simulink model "simulacionesTarea7"  (R2021a)
settings: Solver=VariableStepAuto  StartTime=0.0  StopTime=20  RelTol=1e-3
values from neighbouring files (symbols this model uses):
  A = double(A)    [p1p2.m]    (also in p3.m = [-0.8468   -0.0005;54.4218   -7.6617]; p4Discreto1.m = poly2sym(A, z); p5.m = poly2sym(A, z))
  B = double(B)    [p1p2.m]    (also in p3.m = [0;8.3264]; p4Discreto1.m = poly2sym(B, z); p5.m = poly2sym(B, z))
  C = double(C)    [p1p2.m]    (also in p3.m = [0 1])
  denPID = PIDz.den{1}    [P4.m]
  gdzd = Gd.den{1}    [p4Discreto1.m]    (also in p5.m)
  gdzn = Gd.num{1}    [p4Discreto1.m]    (also in p5.m)
  k1 = eval(Sol.k1)    [p3.m]
  k2 = eval(Sol.k2)    [p3.m]
  kc = double(kc)    [experimentoCompensadores.m]    (also in p5compensador.m)
  kd = eval(S.kd)    [P4.m]
  ki = eval(S.ki)    [P4.m]    (also in p3.m = eval(Sol.ki))
  kp = eval(S.kp)    [P4.m]
  L = [PDO(3)-(6.513); PDO(2)-8.508]    [p3.m]
  numPID = PIDz.num{1}    [P4.m]
  r0 = double(vpa(r0))    [p4Discreto1.m]    (also in p5.m)
  s0 = double(vpa(s0))    [p4Discreto1.m]    (also in p5.m)
  s1 = double(vpa(s1))    [p4Discreto1.m]    (also in p5.m)
  s2 = double(vpa(s2))    [p4Discreto1.m]    (also in p5.m)
  tm = 6/300    (= 0.02)    [P4.m]    (also in p4Discreto1.m; p5.m = 0.125)
  UbiCero = double(UbiCero)    [experimentoCompensadores.m]    (also in p5compensador.m)
  UbiPolo = double(UbiPolo)    [experimentoCompensadores.m]    (also in p5compensador.m)
libraries: simulink x2
settings Model: Creator=Cx001la  LastModifiedBy=Cx001la
settings SolverCC: AlgebraicLoopSolver=TrustRegion
settings DataIOCC: ReturnWorkspaceOutputs=off
settings DebuggingCC: SFMachineParentedDataDiag=warning  ArithmeticOperatorsInVariantConditions=warning
settings SFSimCC: SimUseLocalCustomCode=off  CustomCodeUndefinedFunction=UseInterfaceOnly
settings RTWCC: RTWUseLocalCustomCode=off

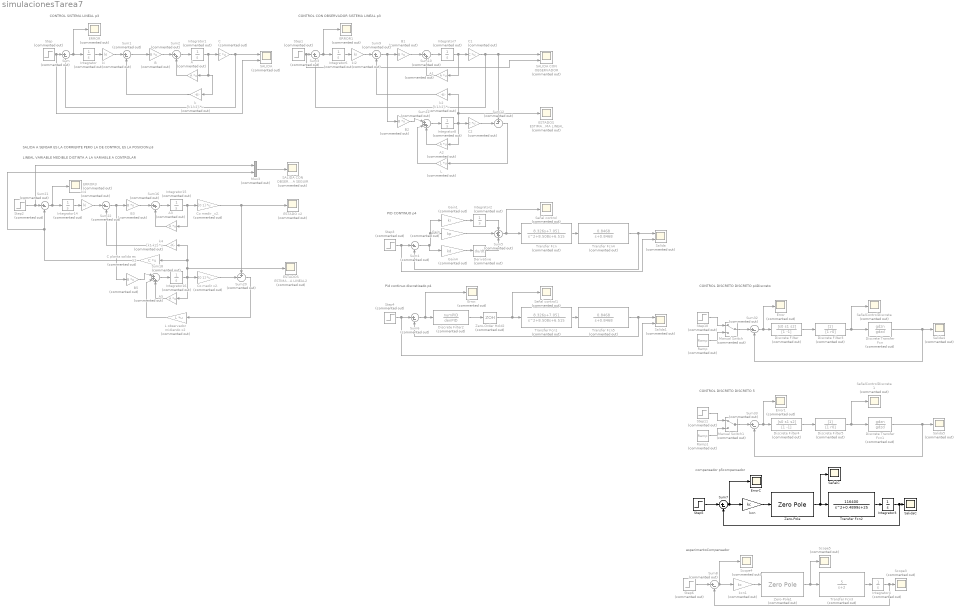
== system simulacionesTarea7 ==
  note: compensador p5compensador
  note: Pid continuo discretizado p4
  note: PID CONTINUO p4
  note: CONTROL SISTEMA LINEAL p3
  note: CONTROL CON OBSERVADOR SISTEMA LINEAL p3
  note: SALIDA A SENSAR ES LA CORRIENTE PERO LA DE CONTROL ES LA POSICION p3
  note: LINEAL VARIABLE MEDIBLE DISTINTA A LA VARIABLE A CONTROLAR
  note: CONTROL DISCRETO DISCRETO p4Discreto
  note: CONTROL DISCRETO DISCRETO 5
  note: esperimentoCompensador
  A{,1..3,5} (5 alike) : Gain  Commented=on  Gain=A  Multiplication=Matrix(K*u)
  B{,1..3,5} (5 alike) : Gain  Commented=on  Gain=B  Multiplication=Matrix(K*u)
  C : Gain  Commented=on  Gain=C  Multiplication=Matrix(K*u)
  C planta salida es X2 : Gain  Commented=on  Gain=C  Multiplication=Matrix(K*u)
  C1 : Gain  Commented=on  Gain=C  Multiplication=Matrix(K*u)
  C2 : Gain  Commented=on  Gain=C  Multiplication=Matrix(K*u)
  Co medir _x2. : Gain  Commented=on  Gain=[0 1]  Multiplication=Matrix(K*u)
  Co medir x2. : Gain  Commented=on  Gain=[0 1]  Multiplication=Matrix(K*u)
  Derivative : Derivative  Commented=on
  Discrete Transfer Fcn : DiscreteTransferFcn  Commented=on  Numerator=gdzn  Denominator=gdzd
  Discrete Transfer Fcn1 : DiscreteTransferFcn  Commented=on  Numerator=gdzn  Denominator=gdzd
  Discrete Filter : DiscreteFilter  Commented=on  Numerator=[s0 s1 s2]  Denominator=[1 -1]
  Discrete Filter2 : DiscreteFilter  Commented=on  Numerator=numPID  Denominator=denPID  SampleTime=tm
  Discrete Filter3 : DiscreteFilter  Commented=on  Denominator=[1 r0]
  Discrete Filter4 : DiscreteFilter  Commented=on  Numerator=[s0 s1 s2]  Denominator=[1 -1]  SampleTime=tm
  Discrete Filter5 : DiscreteFilter  Commented=on  Denominator=[1 r0]  SampleTime=tm
  ERROR : Scope  Commented=on
  ERROR1 : Scope  Commented=on
  ERROR3 : Scope  Commented=on
  ESTADO x2 : Scope  Commented=on
  ESTADOS ESTIMADOS SISTEMA LINEAL : Scope  Commented=on
  ESTADOS ESTIMADOS SISTEMA LINEAL2 : Scope  Commented=on
  Error : Scope  Commented=on
  Error. : Scope  Commented=on
  Error1 : Scope  Commented=on
  ErrorC : Scope
  Gain : Gain  Commented=on  Gain=kp
  Gain1 : Gain  Commented=on  Gain=ki
  Gain4 : Gain  Commented=on  Gain=kd
  Integrator{,1..2,4,6..8,14..16} (10 alike) : Integrator  Commented=on
  Integrator3 : Integrator
  L : Gain  Commented=on  Gain=L  Multiplication=Matrix(K*u)
  L observador midiendo x2 : Gain  Commented=on  Gain=L  Multiplication=Matrix(K*u)
  Manual Switch : ManualSwitch  Commented=on
  Manual Switch1 : ManualSwitch  Commented=on
  Mux3 : Mux  Commented=on  Inputs=2
  Ramp : simulink/Sources/Ramp  Commented=on  slope=1  start=0  InitialOutput=0
  Ramp1 : simulink/Sources/Ramp  Commented=on  slope=1  start=0  InitialOutput=0
  SALIDA : Scope  Commented=on  NumInputPorts=2
  "SALIDA CON OBSERVADOR " : Scope  Commented=on  NumInputPorts=2
  SALIDA CON OBSERVADOR SALIDA ESTIMADA VS REFERENCIA A SEGUIR : Scope  Commented=on
  Salida : Scope  Commented=on  NumInputPorts=2
  Salida1 : Scope  Commented=on  NumInputPorts=2
  Salida4 : Scope  Commented=on
  Salida5 : Scope  Commented=on
  SalidaC : Scope
  Scope3 : Scope  Commented=on
  Scope4 : Scope  Commented=on
  Scope5 : Scope  Commented=on
  Señal control : Scope  Commented=on
  Señal control1 : Scope  Commented=on
  SeñalC : Scope
  SeñalControlDiscreta : Scope  Commented=on
  SeñalControlDiscreta1 : Scope  Commented=on
  Step{,1..2,4,6,11} (6 alike) : Step  Commented=on  Time=0  SampleTime=0
  Step10 : Step  Commented=on  SampleTime=0
  Step3 : Step  Commented=on  SampleTime=0
  Step5 : Step  Time=0  SampleTime=0
  Sum{,1,3..4,6,8..9,21..22,32..33} (11 alike) : Sum  Commented=on  Inputs=|+-
  Sum10 : Sum  Commented=on  Inputs=|++
  Sum11 : Sum  Commented=on  Inputs=|+++
  Sum12 : Sum  Commented=on  Inputs=+-|
  Sum16 : Sum  Commented=on  Inputs=|++
  Sum18 : Sum  Commented=on  Inputs=|+++
  Sum2 : Sum  Commented=on  Inputs=|++
  Sum20 : Sum  Commented=on  Inputs=+-|
  Sum5 : Sum  Commented=on  Inputs=+++
  Sum7 : Sum  Inputs=|+-
  Transfer Fcn : TransferFcn  Commented=on  Numerator=[8.326 7.051]  Denominator=[1 8.508 6.515]
  Transfer Fcn1 : TransferFcn  Commented=on  Numerator=[8.326 7.051]  Denominator=[1 8.508 6.515]
  Transfer Fcn2 : TransferFcn  Numerator=[116400]  Denominator=[1 0.4899 25]
  Transfer Fcn3 : TransferFcn  Commented=on  Numerator=[5]  Denominator=[1 2]
  Transfer Fcn4 : TransferFcn  Commented=on  Numerator=[0.8468]  Denominator=[1 0.8468]
  Transfer Fcn5 : TransferFcn  Commented=on  Numerator=[0.8468]  Denominator=[1 0.8468]
  Zero-Order Hold2 : ZeroOrderHold  Commented=on  SampleTime=tm
  Zero-Pole : ZeroPole  Zeros=[-UbiCero]  Poles=[-UbiPolo]
  Zero-Pole1 : ZeroPole  Commented=on  Zeros=[-UbiCero]  Poles=[-UbiPolo]
  k : Gain  Commented=on  Gain=[k1 k2]  Multiplication=Matrix(K*u)
  k2 : Gain  Commented=on  Gain=[k1 k2]  Multiplication=Matrix(K*u)
  k4 : Gain  Commented=on  Gain=[k1 k2]  Multiplication=Matrix(K*u)
  kcn : Gain  Gain=kc
  kcn1 : Gain  Commented=on  Gain=kc
  ki : Gain  Commented=on  Gain=ki
  ki2 : Gain  Commented=on  Gain=ki
  ki4 : Gain  Commented=on  Gain=ki
  wires:
  C2/1 -> Sum12/2
  Sum3/1 -> ERROR1/1, Integrator6/1
  A/1 -> Sum2/2
  Sum/1 -> ERROR/1, Integrator/1
  Sum12/1 -> L/1
  k2/1 -> Sum9/2
  Integrator7/1 -> A1/1, C1/1
  C1/1 -> Sum12/1, "SALIDA CON OBSERVADOR "/1, Sum3/2
  B2/1 -> Sum11/1
  L/1 -> Sum11/2
  ki2/1 -> Sum9/1
  Integrator6/1 -> ki2/1
  Integrator/1 -> ki/1
  B/1 -> Sum2/1
  Step/1 -> SALIDA/2, Sum/1
  Integrator1/1 -> k/1, A/1, C/1
  k/1 -> Sum1/2
  Sum1/1 -> B/1
  ki/1 -> Sum1/1
  Sum9/1 -> B2/1, B1/1
  Sum10/1 -> Integrator7/1
  B1/1 -> Sum10/1
  C/1 -> SALIDA/1, Sum/2
  Sum11/1 -> Integrator8/1
  A1/1 -> Sum10/2
  Integrator8/1 -> ESTADOS ESTIMADOS SISTEMA LINEAL/1, k2/1, C2/1, A2/1
  A2/1 -> Sum11/3
  Step1/1 -> "SALIDA CON OBSERVADOR "/2, Sum3/1
  Sum2/1 -> Integrator1/1
  Step2/1 -> Mux3/1, Sum21/1
  ki4/1 -> Sum22/1
  C planta salida es X2/1 -> Mux3/2, Sum21/2
  k4/1 -> Sum22/2
  Sum16/1 -> Integrator15/1
  A3/1 -> Sum16/2
  Sum22/1 -> B5/1, B3/1
  B3/1 -> Sum16/1
  A5/1 -> Sum18/3
  B5/1 -> Sum18/1
  L observador midiendo x2/1 -> Sum18/2
  Co medir x2./1 -> Sum20/2
  Sum18/1 -> Integrator16/1
  Mux3/1 -> SALIDA CON OBSERVADOR SALIDA ESTIMADA VS REFERENCIA A SEGUIR/1
  Co medir _x2./1 -> ESTADO x2/1, Sum20/1
  Integrator14/1 -> ki4/1
  Integrator15/1 -> Co medir _x2./1, A3/1
  Sum20/1 -> L observador midiendo x2/1
  Integrator16/1 -> ESTADOS ESTIMADOS SISTEMA LINEAL2/1, k4/1, C planta salida es X2/1, Co medir x2./1, A5/1
  Sum21/1 -> ERROR3/1, Integrator14/1
  Step3/1 -> Salida/2, Sum4/1
  Gain1/1 -> Integrator2/1
  Sum4/1 -> Gain4/1, Gain/1, Gain1/1
  Integrator2/1 -> Sum5/1
  Gain/1 -> Sum5/2
  Sum5/1 -> Señal control/1, Transfer Fcn/1
  Gain4/1 -> Derivative/1
  Derivative/1 -> Sum5/3
  Transfer Fcn/1 -> Transfer Fcn4/1
  Transfer Fcn4/1 -> Sum4/2, Salida/1
  Transfer Fcn5/1 -> Sum6/2, Salida1/1
  Transfer Fcn1/1 -> Transfer Fcn5/1
  Step4/1 -> Salida1/2, Sum6/1
  Sum6/1 -> Error./1, Discrete Filter2/1
  Discrete Filter2/1 -> Zero-Order Hold2/1
  Zero-Order Hold2/1 -> Señal control1/1, Transfer Fcn1/1
  Manual Switch/1 -> Sum32/1
  Ramp/1 -> Manual Switch/2
  Step10/1 -> Manual Switch/1
  Discrete Transfer Fcn/1 -> Salida4/1, Sum32/2
  Sum32/1 -> Error/1, Discrete Filter/1
  Discrete Filter/1 -> Discrete Filter3/1
  Discrete Filter3/1 -> SeñalControlDiscreta/1, Discrete Transfer Fcn/1
  Discrete Filter4/1 -> Discrete Filter5/1
  Sum33/1 -> Error1/1, Discrete Filter4/1
  Discrete Transfer Fcn1/1 -> Salida5/1, Sum33/2
  Discrete Filter5/1 -> SeñalControlDiscreta1/1, Discrete Transfer Fcn1/1
  Step11/1 -> Manual Switch1/1
  Ramp1/1 -> Manual Switch1/2
  Manual Switch1/1 -> Sum33/1
  Step5/1 -> Sum7/1
  Sum7/1 -> ErrorC/1, kcn/1
  kcn/1 -> Zero-Pole/1
  Zero-Pole/1 -> SeñalC/1, Transfer Fcn2/1
  Transfer Fcn2/1 -> Integrator3/1
  Integrator3/1 -> SalidaC/1, Sum7/2
  kcn1/1 -> Zero-Pole1/1
  Integrator4/1 -> Scope3/1, Sum8/2
  Transfer Fcn3/1 -> Integrator4/1
  Zero-Pole1/1 -> Scope5/1, Transfer Fcn3/1
  Step6/1 -> Sum8/1
  Sum8/1 -> Scope4/1, kcn1/1
